simulink model "db4_8zzrb"  (R2018a)
settings: Solver=ode45  StartTime=0.0  StopTime=0.01  MaxStep=3e-5  RelTol=1e-3  AbsTol=1e-3
values from neighbouring files (symbols this model uses):
  fcem = str2num(get(findobj('Tag','variable1'),'String'))    [graficas_a.m]    (also in simulaciones.m = 0)
  Ian = 5    [set_motor.m]
libraries: simulink x2
settings Model: ExtModeTrigMode=oneshot  ExtModeArmWhenConnect=off  Creator=Lac User  LastModifiedBy=Matias
settings SolverCC: AutoScaleAbsTol=off
settings DataIOCC: SaveFormat=Array  SignalLoggingSaveFormat=ModelDataLogs  SaveOutput=off  SaveTime=off
settings OptimizationCC: BlockReduction=off  BooleanDataType=off  LifeSpan=inf
settings DebuggingCC: SaveWithParameterizedLinksMsg=none  UnderspecifiedInitializationDetection=Classic  MergeDetectMultiDrivingBlocksExec=none  SignalResolutionControl=TryResolveAllWithWarning  MultiTaskDSMMsg=warning  MultiTaskCondExecSysMsg=none  SFUnexpectedBacktrackingDiag=warning  SFNoUnconditionalDefaultTransitionDiag=warning  SFExecutionAtInitializationDiag=none
settings HardwareCC: ProdBitPerPointer=32  ProdBitPerSizeT=32  ProdBitPerPtrDiffT=32  ProdLargestAtomicFloat=None  ProdIntDivRoundTo=Undefined  ProdEndianess=Unspecified  ProdWordSize=32  ProdHWDeviceType=32-bit Generic  TargetUnknown=on
settings ModelReferenceCC: PropagateSignalLabelsOutOfModel=off
settings RTWCC: TemplateMakefile=grt_vc.tmf
settings CodeAppCC: StateflowObjectComments=on
settings GRTTargetCC: TargetLangStandard=C89/C90 (ANSI)  GeneratePreprocessorConditionals=Disable all  CombineOutputUpdateFcns=off  GRTInterface=on
settings ConfigComp: CovMetricSettings=dw  CovHtmlReporting=on  CovSaveCumulativeToWorkspaceVar=on  CovSaveSingleToWorkspaceVar=on  CovExternalEMLEnable=off

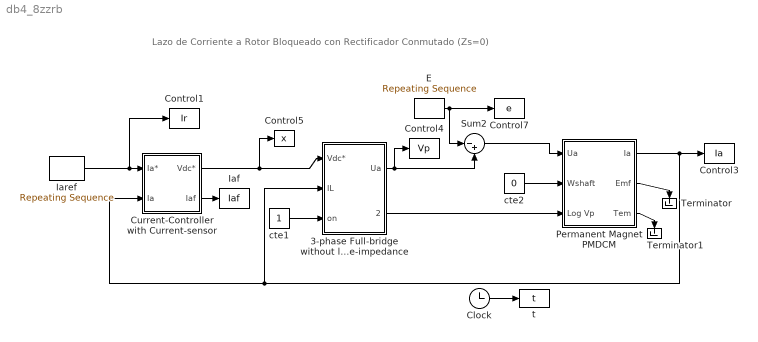
== system db4_8zzrb ==
  note: Lazo de Corriente a Rotor Bloqueado con Rectificador Conmutado (Zs=0)
  3-phase Full-bridge without line-impedance : Subsystem  mask(3-phase Full-bridge without line-impedance){Vph=220, f=50}
      mask prompts: Vph "RMS Phase Voltage [V]:"; f "Frecuency [Hz]:"
      mask init:
      | VLL=(3^.5)*Vph;
  Clock : Clock
  Control1 : ToWorkspace  VariableName=Ir
      settings: MaxDataPoints=200000
  Control3 : ToWorkspace  VariableName=Ia
      settings: MaxDataPoints=200000
  Control4 : ToWorkspace  VariableName=Vp
      settings: MaxDataPoints=200000
  Control5 : ToWorkspace  VariableName=x
      settings: MaxDataPoints=20000
  Control7 : ToWorkspace  VariableName=e
      settings: MaxDataPoints=200000
  Current-Controller with Current-sensor : Subsystem  mask(Current-Controller with Current-sensor){Kpi=0.16, TIi=0.027, Kti=1, Tfi=0.008, VLL=380}
      mask prompts: Kpi "Current Proportional Gain:"; TIi "Current Integral Gain:"; Kti "Current-sensor Proportional Gain:"; Tfi "Current-sensor Integral Gain:"; VLL "RMS Line to Line Voltage [V]:"
  E : simulink/Sources/Repeating Sequence  rep_seq_t="[0   0.6   0.61  0.75   .751   1 ]"  rep_seq_y="[0   0    fcem  fcem  -fcem -fcem]"
  Iaf : ToWorkspace  VariableName=Iaf
      settings: MaxDataPoints=200000
  Iaref : simulink/Sources/Repeating Sequence  rep_seq_t="[0   0.2  0.21    0.35  0.351  0.45  0.451 1]"  rep_seq_y="[Ian Ian  2*Ian 2*Ian  45    45    Ian  Ian]"
  Permanent Magnet PMDCM : Subsystem  mask(Permanent Magnet PMDCM){La=0.003, Ra=0.05, k=6.7851, ic=0}
      mask prompts: La "Armature Inductance  [Hy]:"; Ra "Armature Resistance [Ohms]:"; k "Motor Constant:"; ic "Armature Current Initial Condition [Amp]:"
  Sum2 : Sum  Inputs=|-+  SaturateOnIntegerOverflow=on  InputSameDT=on  OutDataTypeStr=Inherit: Same as first input
  Terminator : Terminator
  Terminator1 : Terminator
  cte1 : Constant
  cte2 : Constant  Value=0
  t : ToWorkspace  VariableName=t
      settings: MaxDataPoints=200000
  wires:
  cte1/1 -> 3-phase Full-bridge without line-impedance/3(on)
  Iaref/1 -> Control1/1, Current-Controller with Current-sensor/1(Ia*)
  Current-Controller with Current-sensor/1(Vdc*) -> Control5/1, 3-phase Full-bridge without line-impedance/1(Vdc*)
  Current-Controller with Current-sensor/2(Iaf) -> Iaf/1
  Clock/1 -> t/1
  3-phase Full-bridge without line-impedance/1(Ua) -> Control4/1, Sum2/2
  Permanent Magnet PMDCM/1(Ia) -> Control3/1, 3-phase Full-bridge without line-impedance/2(IL), Current-Controller with Current-sensor/2(Ia)
  3-phase Full-bridge without line-impedance/2(log Ua) -> Permanent Magnet PMDCM/3(Log Vp)
  Sum2/1 -> Permanent Magnet PMDCM/1(Ua)
  E/1 -> Sum2/1, Control7/1
  cte2/1 -> Permanent Magnet PMDCM/2(Wshaft)
  Permanent Magnet PMDCM/2(Emf) -> Terminator/1
  Permanent Magnet PMDCM/3(Tem) -> Terminator1/1

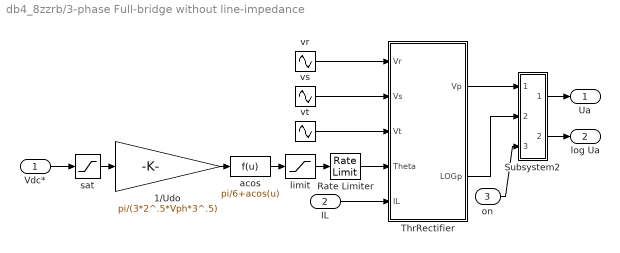
== system db4_8zzrb/3-phase Full-bridge without line-impedance ==
  Vdc* : Inport
  IL : Inport  Port=2
  on : Inport  Port=3
  1/Udo : Gain  Gain=pi/(3*2^.5*Vph*3^.5)  SaturateOnIntegerOverflow=on  OutDataTypeStr=Inherit: Same as input  ParamDataTypeStr=Inherit: Same as input
  Rate Limiter : RateLimiter  RisingSlewLimit=8000  FallingSlewLimit=-8000
  Subsystem2 : Subsystem
  ThrRectifier : Subsystem
      mask Display:
      | plot([0.3 0.7 0.5 0.3],[0.4 0.4 0.6 0.4])
      | plot([0.3 0.7 ],[0.6 0.6])
      | plot([0.5 0.5 ],[0.6 0.7])
      | plot([0.5 0.5 ],[0.3 0.4])
      | plot([0.35 0.5],[0.7 0.6])
      | plot([0.25 0.35 ],[0.7 0.7])
  acos : Fcn  Expr=pi/6+acos(u)
  limit : Saturate  UpperLimit=pi*6.999/6  LowerLimit=pi/5.998
  sat : Saturate  UpperLimit=(3*2^.5*3^.5*Vph)/pi  LowerLimit=-((3*2^.5*3^.5*Vph)/pi)
  vr : Sin  Amplitude=Vph*(2^.5)  Frequency=2*pi*f  SampleTime=0
  vs : Sin  Amplitude=Vph*(2^.5)  Frequency=2*pi*f  Phase=-(2/3)*pi  SampleTime=0
  vt : Sin  Amplitude=Vph*(2^.5)  Frequency=2*pi*f  Phase=-(4/3)*pi  SampleTime=0
  Ua : Outport
  log Ua : Outport  Port=2
  wires:
  Rate Limiter/1 -> ThrRectifier/4(Theta)
  IL/1 -> ThrRectifier/5(IL)
  vt/1 -> ThrRectifier/3(Vt)
  on/1 -> Subsystem2/3(in_2)
  Subsystem2/2(out_2) -> log Ua/1
  Vdc*/1 -> sat/1
  Subsystem2/1(out_1) -> Ua/1
  ThrRectifier/1(Vp) -> Subsystem2/1(in_1)
  limit/1 -> Rate Limiter/1
  ThrRectifier/2(LOGp) -> Subsystem2/2(in_3)
  vs/1 -> ThrRectifier/2(Vs)
  vr/1 -> ThrRectifier/1(Vr)
  1/Udo/1 -> acos/1
  acos/1 -> limit/1
  sat/1 -> 1/Udo/1

== system db4_8zzrb/Current-Controller with Current-sensor ==
  Ia* : Inport
  Ia : Inport  Port=2
  Ftr : TransferFcn  Numerator=[Kti]  Denominator=[Tfi 1]
  I - Ctr : Subsystem
      mask Display: plot([0 .01  5],[0 2 4])
  Sum1 : Sum  Inputs=+-  SaturateOnIntegerOverflow=on  InputSameDT=on  OutDataTypeStr=Inherit: Same as first input
  Vdc* : Outport
  Iaf : Outport  Port=2
  wires:
  Ia*/1 -> Sum1/1
  Ia/1 -> Ftr/1, I - Ctr/2(Ia)
  Sum1/1 -> I - Ctr/1(Ia*- Iaf)
  I - Ctr/1(Vd*) -> Vdc*/1
  Ftr/1 -> Sum1/2, Iaf/1

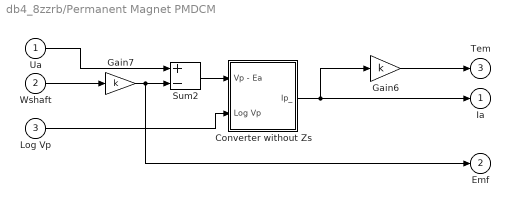
== system db4_8zzrb/Permanent Magnet PMDCM ==
  Ua : Inport
  Wshaft : Inport  Port=2
  Log Vp : Inport  Port=3
  Converter without Zs : Subsystem
  Gain6 : Gain  Gain=k  SaturateOnIntegerOverflow=on  OutDataTypeStr=Inherit: Same as input  ParamDataTypeStr=Inherit: Same as input
  Gain7 : Gain  Gain=k  SaturateOnIntegerOverflow=on  OutDataTypeStr=Inherit: Same as input  ParamDataTypeStr=Inherit: Same as input
  Sum2 : Sum  Inputs=+-  SaturateOnIntegerOverflow=on  InputSameDT=on  OutDataTypeStr=Inherit: Same as first input
  Ia : Outport
  Emf : Outport  Port=2
  Tem : Outport  Port=3
  wires:
  Wshaft/1 -> Gain7/1
  Ua/1 -> Sum2/1
  Sum2/1 -> Converter without Zs/1(Vp - Ea)
  Gain7/1 -> Sum2/2, Emf/1
  Log Vp/1 -> Converter without Zs/2(Log Vp)
  Converter without Zs/1(Ip_) -> Ia/1, Gain6/1
  Gain6/1 -> Tem/1

== system db4_8zzrb/3-phase Full-bridge without line-impedance/Subsystem2 ==
  in_1 : Inport
  in_3 : Inport  Port=2
  in_2 : Inport  Port=3
  Product1 : Product  SaturateOnIntegerOverflow=on  RndMeth=Zero  InputSameDT=on  OutDataTypeStr=Inherit: Same as first input
  Product2 : Product  SaturateOnIntegerOverflow=on  RndMeth=Zero  InputSameDT=on  OutDataTypeStr=Inherit: Same as first input
  out_1 : Outport
  out_2 : Outport  Port=2
  wires:
  in_3/1 -> Product2/2
  in_2/1 -> Product2/1, Product1/2
  Product2/1 -> out_2/1
  Product1/1 -> out_1/1
  in_1/1 -> Product1/1

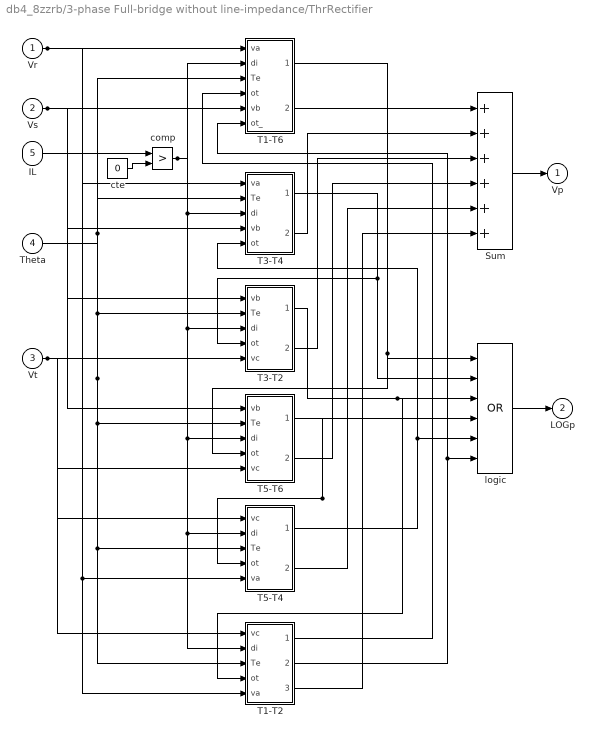
== system db4_8zzrb/3-phase Full-bridge without line-impedance/ThrRectifier ==
  Vr : Inport
  Vs : Inport  Port=2
  Vt : Inport  Port=3
  Theta : Inport  Port=4
  IL : Inport  Port=5
  Sum : Sum  Inputs=++++++  SaturateOnIntegerOverflow=on  InputSameDT=on  OutDataTypeStr=Inherit: Same as first input
  T1-T2 : Subsystem
  T1-T6 : Subsystem
  T3-T2 : Subsystem
  T3-T4 : Subsystem
  T5-T4 : Subsystem
  T5-T6 : Subsystem
  comp : RelationalOperator  Operator=>  RndMeth=Nearest  InputSameDT=on
  cte : Constant  Value=0
  logic : Logic  Operator=OR  Inputs=6
  Vp : Outport
  LOGp : Outport  Port=2
  wires:
  T3-T2/2(out_2) -> Sum/3
  Vr/1 -> T1-T6/1(va), T3-T4/1(va), T5-T4/5(va), T1-T2/5(va)
  Vs/1 -> T3-T4/4(vb), T5-T6/1(vb), T3-T2/1(vb), T1-T6/5(vb)
  Vt/1 -> T5-T6/5(vc), T1-T2/1(vc), T5-T4/1(vc), T3-T2/5(vc)
  comp/1 -> T1-T6/2(di), T3-T4/3(di), T3-T2/3(di), T5-T6/3(di), T5-T4/2(di), T1-T2/2(di)
  T1-T6/2(out_2) -> Sum/1
  T3-T4/2(out_2) -> Sum/2
  T1-T2/1(out_1) -> T1-T6/4(ot)
  T5-T6/2(out_2) -> Sum/4
  T5-T4/2(out_2) -> Sum/5
  T1-T2/3(out_3) -> Sum/6
  T5-T6/1(out_1) -> logic/4, T5-T4/4(ot)
  T1-T6/1(out_1) -> T5-T6/4(ot), logic/1
  logic/1 -> LOGp/1
  Sum/1 -> Vp/1
  cte/1 -> comp/2
  IL/1 -> comp/1
  T3-T4/1(out_1) -> T3-T2/4(ot), logic/2
  Theta/1 -> T3-T2/2(Te), T1-T6/3(Te), T3-T4/2(Te), T5-T4/3(Te), T1-T2/3(Te), T5-T6/2(Te)
  T5-T4/1(out_1) -> logic/5, T3-T4/5(ot)
  T1-T2/2(out_2) -> logic/6, T1-T6/6(ot_)
  T3-T2/1(out_1) -> logic/3, T1-T2/4(ot)

== system db4_8zzrb/Current-Controller with Current-sensor/I - Ctr ==
  Ia*- Iaf : Inport
  Ia : Inport  Port=2
  Adaptative Control : Subsystem
  comp : RelationalOperator  Operator=>  RndMeth=Nearest  InputSameDT=on
  cte1 : Constant  Value=0
  sat : Saturate  UpperLimit=VLL*sqrt(2)*3/pi  LowerLimit=-VLL*sqrt(2)*3/pi
  Vd* : Outport
  wires:
  Ia*- Iaf/1 -> Adaptative Control/2(Ia*- Iaf)
  cte1/1 -> comp/2
  sat/1 -> Vd*/1
  Adaptative Control/1(Vd*) -> sat/1
  comp/1 -> Adaptative Control/1(Ia>0)
  Ia/1 -> comp/1

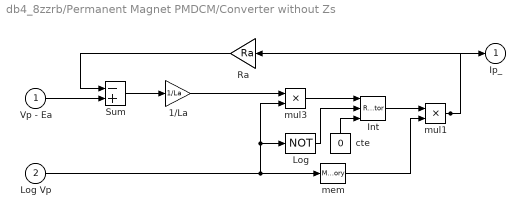
== system db4_8zzrb/Permanent Magnet PMDCM/Converter without Zs ==
  Vp - Ea : Inport
  Log Vp : Inport  Port=2
  1/La : Gain  Gain=1/La  SaturateOnIntegerOverflow=on  OutDataTypeStr=Inherit: Same as input  ParamDataTypeStr=Inherit: Same as input
  Int : ResetIntegrator
  Log : Logic  Operator=NOT  Inputs=1
  Ra : Gain  Gain=Ra  SaturateOnIntegerOverflow=on  OutDataTypeStr=Inherit: Same as input  ParamDataTypeStr=Inherit: Same as input
  Sum : Sum  Inputs=-+  SaturateOnIntegerOverflow=on  InputSameDT=on  OutDataTypeStr=Inherit: Same as first input
  cte : Constant  Value=0
  mem : Memory
  mul1 : Product  SaturateOnIntegerOverflow=on  RndMeth=Zero  InputSameDT=on  OutDataTypeStr=Inherit: Same as first input
  mul3 : Product  SaturateOnIntegerOverflow=on  RndMeth=Zero  InputSameDT=on  OutDataTypeStr=Inherit: Same as first input
  Ip_ : Outport
  wires:
  Ra/1 -> Sum/1
  Vp - Ea/1 -> Sum/2
  1/La/1 -> mul3/1
  mul1/1 -> Ip_/1, Ra/1
  cte/1 -> Int/3
  Log/1 -> Int/2
  mul3/1 -> Int/1
  Int/1 -> mul1/1
  mem/1 -> mul1/2
  Sum/1 -> 1/La/1
  Log Vp/1 -> Log/1, mul3/2, mem/1

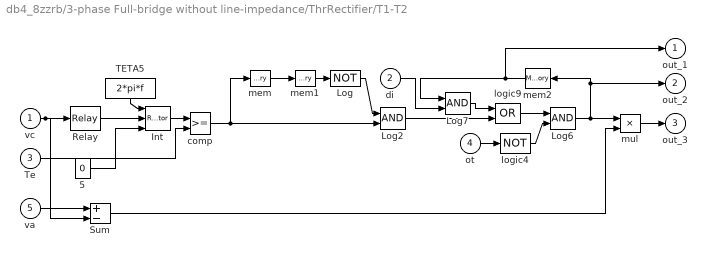
== system db4_8zzrb/3-phase Full-bridge without line-impedance/ThrRectifier/T1-T2 ==
  vc : Inport
  di : Inport  Port=2
  Te : Inport  Port=3
  ot : Inport  Port=4
  va : Inport  Port=5
  5 : Constant  Value=0
  Int : ResetIntegrator
  Log : Logic  Operator=NOT  Inputs=1
  Log2 : Logic
  Log6 : Logic
  Log7 : Logic
  Relay : Relay  OnSwitchValue=(2^.5)*Vph*sin(pi/6)  OffSwitchValue=0
  Sum : Sum  Inputs=+-  SaturateOnIntegerOverflow=on  InputSameDT=on  OutDataTypeStr=Inherit: Same as first input
  TETA5 : Constant  Value=2*pi*f
  comp : RelationalOperator  RndMeth=Nearest  InputSameDT=on
  logic4 : Logic  Operator=NOT  Inputs=1
  logic9 : Logic  Operator=OR
  mem : Memory
  mem1 : Memory
  mem2 : Memory
  mul : Product  SaturateOnIntegerOverflow=on  RndMeth=Zero  InputSameDT=on  OutDataTypeStr=Inherit: Same as first input
  out_1 : Outport
  out_2 : Outport  Port=2
  out_3 : Outport  Port=3
  wires:
  di/1 -> Log7/2
  logic4/1 -> Log6/2
  Log6/1 -> out_2/1, mem2/1, mul/1
  mem2/1 -> out_1/1, Log7/1
  logic9/1 -> Log6/1
  Log7/1 -> logic9/1
  Log2/1 -> logic9/2
  Sum/1 -> mul/2
  5/1 -> Int/3
  TETA5/1 -> Int/1
  Int/1 -> comp/1
  Te/1 -> comp/2
  mul/1 -> out_3/1
  ot/1 -> logic4/1
  va/1 -> Sum/1
  vc/1 -> Sum/2, Relay/1
  Relay/1 -> Int/2
  mem1/1 -> Log/1
  mem/1 -> mem1/1
  Log/1 -> Log2/1
  comp/1 -> mem/1, Log2/2

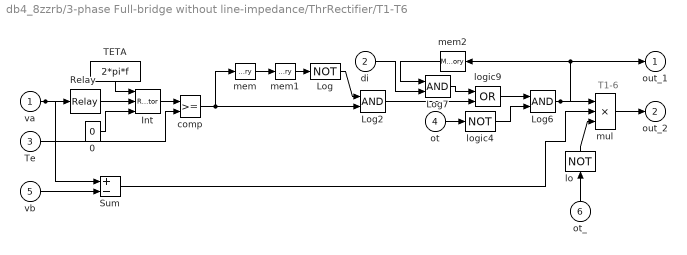
== system db4_8zzrb/3-phase Full-bridge without line-impedance/ThrRectifier/T1-T6 ==
  note: T1-6
  va : Inport
  di : Inport  Port=2
  Te : Inport  Port=3
  ot : Inport  Port=4
  vb : Inport  Port=5
  ot_ : Inport  Port=6
  0 : Constant  Value=0
  Int : ResetIntegrator
  Log : Logic  Operator=NOT  Inputs=1
  Log2 : Logic
  Log6 : Logic
  Log7 : Logic
  Relay : Relay  OnSwitchValue=0  OffSwitchValue=(2^.5)*Vph*sin(pi/6+pi)  OnOutputValue=0  OffOutputValue=1
  Sum : Sum  Inputs=+-  SaturateOnIntegerOverflow=on  InputSameDT=on  OutDataTypeStr=Inherit: Same as first input
  TETA : Constant  Value=2*pi*f
  comp : RelationalOperator  RndMeth=Nearest  InputSameDT=on
  lo : Logic  Operator=NOT  Inputs=1
  logic4 : Logic  Operator=NOT  Inputs=1
  logic9 : Logic  Operator=OR
  mem : Memory
  mem1 : Memory
  mem2 : Memory
  mul : Product  Inputs=3  SaturateOnIntegerOverflow=on  RndMeth=Zero  InputSameDT=on  OutDataTypeStr=Inherit: Same as first input
  out_1 : Outport
  out_2 : Outport  Port=2
  wires:
  Log6/1 -> mul/1, mem2/1, out_1/1
  di/1 -> Log7/2
  logic4/1 -> Log6/2
  logic9/1 -> Log6/1
  Log7/1 -> logic9/1
  mem2/1 -> Log7/1
  Log2/1 -> logic9/2
  lo/1 -> mul/3
  Log/1 -> Log2/1
  0/1 -> Int/3
  Sum/1 -> mul/2
  TETA/1 -> Int/1
  Int/1 -> comp/1
  va/1 -> Relay/1, Sum/1
  Te/1 -> comp/2
  mul/1 -> out_2/1
  ot/1 -> logic4/1
  vb/1 -> Sum/2
  ot_/1 -> lo/1
  Relay/1 -> Int/2
  mem1/1 -> Log/1
  mem/1 -> mem1/1
  comp/1 -> Log2/2, mem/1

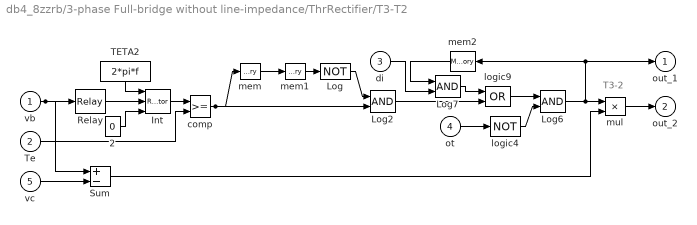
== system db4_8zzrb/3-phase Full-bridge without line-impedance/ThrRectifier/T3-T2 ==
  note: T3-2
  vb : Inport
  Te : Inport  Port=2
  di : Inport  Port=3
  ot : Inport  Port=4
  vc : Inport  Port=5
  2 : Constant  Value=0
  Int : ResetIntegrator
  Log : Logic  Operator=NOT  Inputs=1
  Log2 : Logic
  Log6 : Logic
  Log7 : Logic
  Relay : Relay  OnSwitchValue=0  OffSwitchValue=(2^.5)*Vph*sin(pi/6+pi)  OnOutputValue=0  OffOutputValue=1
  Sum : Sum  Inputs=+-  SaturateOnIntegerOverflow=on  InputSameDT=on  OutDataTypeStr=Inherit: Same as first input
  TETA2 : Constant  Value=2*pi*f
  comp : RelationalOperator  RndMeth=Nearest  InputSameDT=on
  logic4 : Logic  Operator=NOT  Inputs=1
  logic9 : Logic  Operator=OR
  mem : Memory
  mem1 : Memory
  mem2 : Memory
  mul : Product  SaturateOnIntegerOverflow=on  RndMeth=Zero  InputSameDT=on  OutDataTypeStr=Inherit: Same as first input
  out_1 : Outport
  out_2 : Outport  Port=2
  wires:
  Log6/1 -> mem2/1, out_1/1, mul/1
  di/1 -> Log7/2
  logic4/1 -> Log6/2
  logic9/1 -> Log6/1
  Log7/1 -> logic9/1
  mem2/1 -> Log7/1
  Log2/1 -> logic9/2
  Sum/1 -> mul/2
  2/1 -> Int/3
  TETA2/1 -> Int/1
  Relay/1 -> Int/2
  Int/1 -> comp/1
  Te/1 -> comp/2
  mul/1 -> out_2/1
  ot/1 -> logic4/1
  vc/1 -> Sum/2
  vb/1 -> Sum/1, Relay/1
  mem1/1 -> Log/1
  mem/1 -> mem1/1
  Log/1 -> Log2/1
  comp/1 -> Log2/2, mem/1

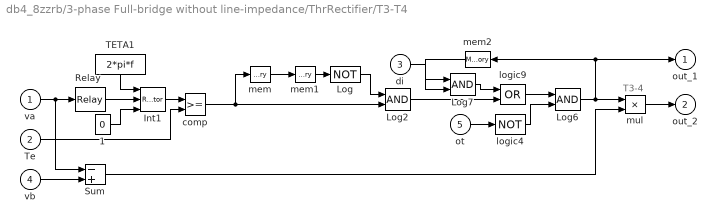
== system db4_8zzrb/3-phase Full-bridge without line-impedance/ThrRectifier/T3-T4 ==
  note: T3-4
  va : Inport
  Te : Inport  Port=2
  di : Inport  Port=3
  vb : Inport  Port=4
  ot : Inport  Port=5
  1 : Constant  Value=0
  Int1 : ResetIntegrator  InitialCondition=pi
  Log : Logic  Operator=NOT  Inputs=1
  Log2 : Logic
  Log6 : Logic
  Log7 : Logic
  Relay : Relay  OnSwitchValue=(2^.5)*Vph*sin(pi/6)  OffSwitchValue=0
  Sum : Sum  Inputs=-+  SaturateOnIntegerOverflow=on  InputSameDT=on  OutDataTypeStr=Inherit: Same as first input
  TETA1 : Constant  Value=2*pi*f
  comp : RelationalOperator  RndMeth=Nearest  InputSameDT=on
  logic4 : Logic  Operator=NOT  Inputs=1
  logic9 : Logic  Operator=OR
  mem : Memory
  mem1 : Memory
  mem2 : Memory
  mul : Product  SaturateOnIntegerOverflow=on  RndMeth=Zero  InputSameDT=on  OutDataTypeStr=Inherit: Same as first input
  out_1 : Outport
  out_2 : Outport  Port=2
  wires:
  Log6/1 -> mem2/1, out_1/1, mul/1
  logic4/1 -> Log6/2
  di/1 -> Log7/2
  logic9/1 -> Log6/1
  Log7/1 -> logic9/1
  mem2/1 -> Log7/1
  Log2/1 -> logic9/2
  comp/1 -> Log2/2, mem/1
  Log/1 -> Log2/1
  1/1 -> Int1/3
  TETA1/1 -> Int1/1
  Int1/1 -> comp/1
  Te/1 -> comp/2
  mul/1 -> out_2/1
  ot/1 -> logic4/1
  Relay/1 -> Int1/2
  mem1/1 -> Log/1
  mem/1 -> mem1/1
  va/1 -> Sum/1, Relay/1
  vb/1 -> Sum/2
  Sum/1 -> mul/2

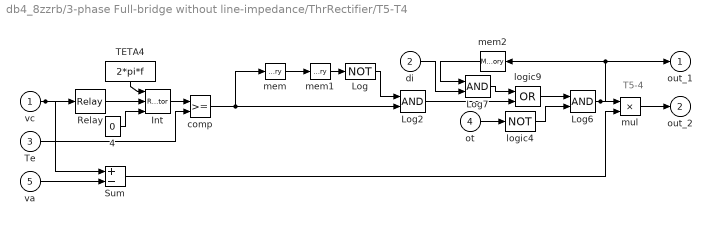
== system db4_8zzrb/3-phase Full-bridge without line-impedance/ThrRectifier/T5-T4 ==
  note: T5-4
  vc : Inport
  di : Inport  Port=2
  Te : Inport  Port=3
  ot : Inport  Port=4
  va : Inport  Port=5
  4 : Constant  Value=0
  Int : ResetIntegrator  InitialCondition=2/3*pi
  Log : Logic  Operator=NOT  Inputs=1
  Log2 : Logic
  Log6 : Logic
  Log7 : Logic
  Relay : Relay  OnSwitchValue=0  OffSwitchValue=(2^.5)*Vph*sin(pi/6+pi)  OnOutputValue=0  OffOutputValue=1
  Sum : Sum  Inputs=+-  SaturateOnIntegerOverflow=on  InputSameDT=on  OutDataTypeStr=Inherit: Same as first input
  TETA4 : Constant  Value=2*pi*f
  comp : RelationalOperator  RndMeth=Nearest  InputSameDT=on
  logic4 : Logic  Operator=NOT  Inputs=1
  logic9 : Logic  Operator=OR
  mem : Memory
  mem1 : Memory
  mem2 : Memory
  mul : Product  SaturateOnIntegerOverflow=on  RndMeth=Zero  InputSameDT=on  OutDataTypeStr=Inherit: Same as first input
  out_1 : Outport
  out_2 : Outport  Port=2
  wires:
  di/1 -> Log7/2
  logic4/1 -> Log6/2
  Log6/1 -> mul/1, mem2/1, out_1/1
  logic9/1 -> Log6/1
  Log7/1 -> logic9/1
  mem2/1 -> Log7/1
  Log2/1 -> logic9/2
  Sum/1 -> mul/2
  4/1 -> Int/3
  TETA4/1 -> Int/1
  Int/1 -> comp/1
  Te/1 -> comp/2
  mul/1 -> out_2/1
  ot/1 -> logic4/1
  va/1 -> Sum/2
  vc/1 -> Sum/1, Relay/1
  Relay/1 -> Int/2
  mem1/1 -> Log/1
  mem/1 -> mem1/1
  Log/1 -> Log2/1
  comp/1 -> mem/1, Log2/2

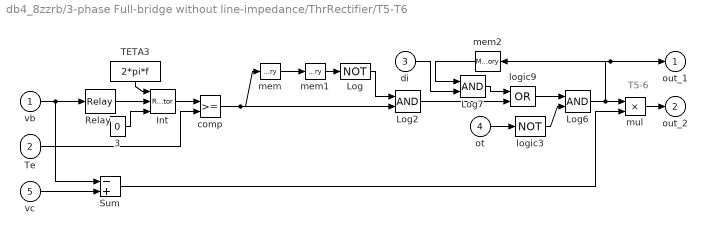
== system db4_8zzrb/3-phase Full-bridge without line-impedance/ThrRectifier/T5-T6 ==
  note: T5-6
  vb : Inport
  Te : Inport  Port=2
  di : Inport  Port=3
  ot : Inport  Port=4
  vc : Inport  Port=5
  3 : Constant  Value=0
  Int : ResetIntegrator  InitialCondition=pi/3
  Log : Logic  Operator=NOT  Inputs=1
  Log2 : Logic
  Log6 : Logic
  Log7 : Logic
  Relay : Relay  OnSwitchValue=(2^.5)*Vph*sin(pi/6)  OffSwitchValue=0
  Sum : Sum  Inputs=-+  SaturateOnIntegerOverflow=on  InputSameDT=on  OutDataTypeStr=Inherit: Same as first input
  TETA3 : Constant  Value=2*pi*f
  comp : RelationalOperator  RndMeth=Nearest  InputSameDT=on
  logic3 : Logic  Operator=NOT  Inputs=1
  logic9 : Logic  Operator=OR
  mem : Memory
  mem1 : Memory
  mem2 : Memory
  mul : Product  SaturateOnIntegerOverflow=on  RndMeth=Zero  InputSameDT=on  OutDataTypeStr=Inherit: Same as first input
  out_1 : Outport
  out_2 : Outport  Port=2
  wires:
  di/1 -> Log7/2
  logic3/1 -> Log6/2
  Log6/1 -> mem2/1, out_1/1, mul/1
  logic9/1 -> Log6/1
  Log7/1 -> logic9/1
  mem2/1 -> Log7/1
  Log2/1 -> logic9/2
  Sum/1 -> mul/2
  3/1 -> Int/3
  TETA3/1 -> Int/1
  Int/1 -> comp/1
  Te/1 -> comp/2
  mul/1 -> out_2/1
  ot/1 -> logic3/1
  Relay/1 -> Int/2
  mem1/1 -> Log/1
  mem/1 -> mem1/1
  Log/1 -> Log2/1
  comp/1 -> Log2/2, mem/1
  vc/1 -> Sum/2
  vb/1 -> Sum/1, Relay/1

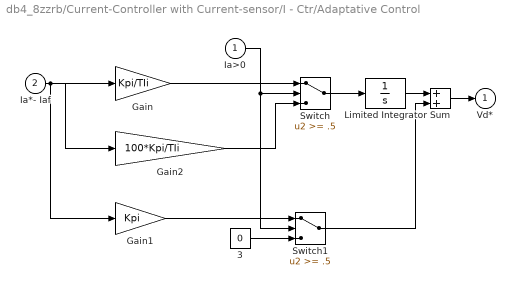
== system db4_8zzrb/Current-Controller with Current-sensor/I - Ctr/Adaptative Control ==
  Ia>0 : Inport
  Ia*- Iaf : Inport  Port=2
  3 : Constant  Value=0
  Gain : Gain  Gain=Kpi/TIi  SaturateOnIntegerOverflow=on  OutDataTypeStr=Inherit: Same as input  ParamDataTypeStr=Inherit: Same as input
  Gain1 : Gain  Gain=Kpi  SaturateOnIntegerOverflow=on  OutDataTypeStr=Inherit: Same as input  ParamDataTypeStr=Inherit: Same as input
  Gain2 : Gain  Gain=100*Kpi/TIi  SaturateOnIntegerOverflow=on  OutDataTypeStr=Inherit: Same as input  ParamDataTypeStr=Inherit: Same as input
  Limited Integrator : Integrator  LimitOutput=on  UpperSaturationLimit=VLL*sqrt(2)*3/pi  LowerSaturationLimit=-VLL*sqrt(2)*3/pi
  Sum : Sum  SaturateOnIntegerOverflow=on  InputSameDT=on  OutDataTypeStr=Inherit: Same as first input
  Switch : Switch  Threshold=.5  SaturateOnIntegerOverflow=on  InputSameDT=on
  Switch1 : Switch  Threshold=.5  SaturateOnIntegerOverflow=on  InputSameDT=on
  Vd* : Outport
  wires:
  Ia>0/1 -> Switch1/2, Switch/2
  3/1 -> Switch1/3
  Gain1/1 -> Switch1/1
  Gain2/1 -> Switch/3
  Switch/1 -> Limited Integrator/1
  Gain/1 -> Switch/1
  Ia*- Iaf/1 -> Gain2/1, Gain1/1, Gain/1
  Sum/1 -> Vd*/1
  Limited Integrator/1 -> Sum/1
  Switch1/1 -> Sum/2
